simulink model "model_sled_syst"  (R2021b)
settings: Solver=ode45  StartTime=0.0  StopTime=0.5  RelTol=1e-3  EnableMultiTasking=on
libraries: simulink x1
settings Model: Creator=Алекс  LastModifiedBy=Admin
settings SolverCC: AlgebraicLoopSolver=TrustRegion
settings DataIOCC: LimitDataPoints=on  SaveFormat=Array  SignalLoggingSaveFormat=ModelDataLogs  ReturnWorkspaceOutputs=off
settings OptimizationCC: ExpressionDepthLimit=2147483647  LifeSpan=inf
settings DebuggingCC: UnderspecifiedInitializationDetection=Classic  MergeDetectMultiDrivingBlocksExec=none  SolverPrmCheckMsg=warning  FcnCallInpInsideContextMsg=warning  StateNameClashWarn=warning  SFUnexpectedBacktrackingDiag=warning  SFNoUnconditionalDefaultTransitionDiag=warning  SFExecutionAtInitializationDiag=none  SFMachineParentedDataDiag=warning  ArithmeticOperatorsInVariantConditions=warning
settings HardwareCC: ProdBitPerPointer=32  ProdBitPerSizeT=32  ProdBitPerPtrDiffT=32  ProdLargestAtomicFloat=None  ProdIntDivRoundTo=Undefined  ProdEndianess=Unspecified  ProdWordSize=32  ProdHWDeviceType=32-bit Generic
settings ModelReferenceCC: PropagateSignalLabelsOutOfModel=off
settings SFSimCC: SimUseLocalCustomCode=off  CustomCodeUndefinedFunction=UseInterfaceOnly
settings RTWCC: RTWUseLocalCustomCode=off
settings CodeAppCC: StateflowObjectComments=on
settings GRTTargetCC: TargetLangStandard=C89/C90 (ANSI)  CombineOutputUpdateFcns=off  GRTInterface=on
settings ConfigComp: CovMetricSettings=dw  CovSaveCumulativeToWorkspaceVar=on  CovSaveSingleToWorkspaceVar=on  CovExternalEMLEnable=off

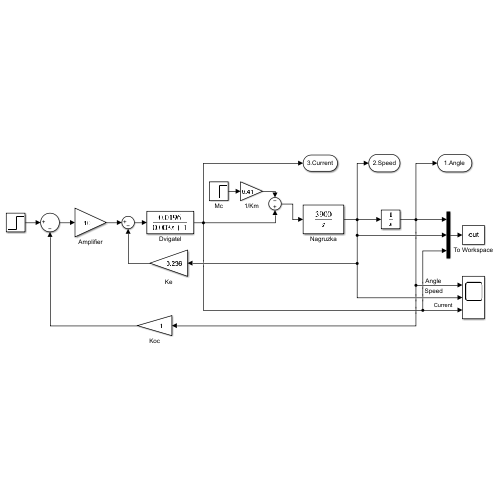
[thumbnail: Simulink's stored preview of the top-level diagram]
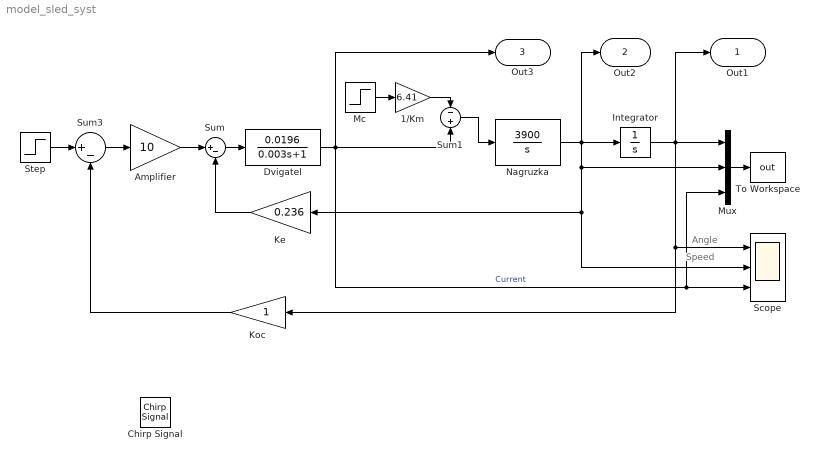
== system model_sled_syst ==
  note: Angle
  note: Speed
  1/Km : Gain  Gain=6.41
  Amplifier : Gain  Gain=10
  Dvigatel : TransferFcn  Numerator=[0.0196]  Denominator=[0.003 1]
  Integrator : Integrator
  Ke : Gain  Gain=0.236
  Koc : Gain
  Mc : Step  Time=0  After=0  SampleTime=0
  Mux : Mux  Inputs=3
  Nagruzka : TransferFcn  Numerator=[3900]  Denominator=[1 0]
  Scope : Scope  NumInputPorts=3
      settings: RequirementInfo={} %GIDa_d75e19c9_9626_491c_be70_c8873396050c
  Step : Step  Time=0  SampleTime=0  VectorParams1D=off  ZeroCross=off
  Sum : Sum  Inputs=|+-
  Sum1 : Sum  Inputs=-+
  Sum3 : Sum  Inputs=|+-
  To Workspace : ToWorkspace  VariableName=out  SampleTime=1e-5
  Out1 : Outport  BusOutputAsStruct=on
  Out2 : Outport  Port=2  BusOutputAsStruct=on
  Out3 : Outport  Port=3  BusOutputAsStruct=on
  Chirp Signal : simulink/Sources/Chirp Signal  IOType=siggen  f1=0.1  T=100  f2=1
  wires:
  Sum/1 -> Dvigatel/1
  Nagruzka/1 -> Ke/1, Scope/2, Mux/2, Out2/1, Integrator/1
  Ke/1 -> Sum/2
  Integrator/1 -> Out1/1, Mux/1, Koc/1, Scope/1
  Mux/1 -> To Workspace/1
  Koc/1 -> Sum3/2
  Dvigatel/1 -> Scope/3, Mux/3, Sum1/2, Out3/1  "Current"
  Sum1/1 -> Nagruzka/1
  1/Km/1 -> Sum1/1
  Amplifier/1 -> Sum/1
  Sum3/1 -> Amplifier/1
  Mc/1 -> 1/Km/1
  Step/1 -> Sum3/1
